simulink model "Citation_Sim"  (R2019b)
settings: Solver=VariableStepAuto  StartTime=0.0  StopTime=10.0  RelTol=1e-3
values from neighbouring files (symbols this model uses):
  A = [-0.0151 -60.5651 0 -32.174 ... (first row only)    [UnstableAircraft.m]    (also in VincentMPCCode.m = [0 0 1 0; 0 0 0 1; -(Ks+Kus)/Mus Ks/Mus -Bs/Mus Bs/Mus; Ks/M; qpsoft.m = [           A,             minusones; scmpc4.m = [A;Su(iymax,:)]; scmpcnl2.m = [A;Su(iymax,:)])
  B = [-2.516 -13.136 ... (first row only)    [UnstableAircraft.m]    (also in VincentMPCCode.m = [0 0; 0 0; -1/Mus Kus/Mus; 1/Ms 0]; qpsoft.m = [         B; scmpc4.m = SuTQ*Su+diag(R); scmpcnl2.m = SuTQ*Su+diag(R))
  C = [0 1 0 0 ... (first row only)    [UnstableAircraft.m]    (also in VincentMPCCode.m = [1 0 0 0; -1 1 0 0; 0 0 1 0; 0 0 0 1])
  D = [0 0 ... (first row only)    [UnstableAircraft.m]    (also in VincentMPCCode.m = [0 -1; 0 0; 0 0; 0 0])
libraries: mpclib x1
settings Model: Creator=kieran  LastModifiedBy=kieran

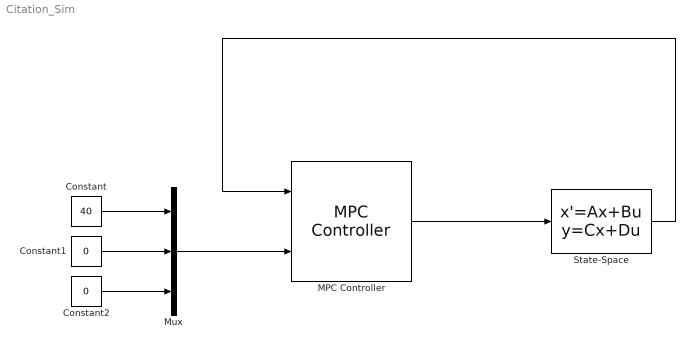
== system Citation_Sim ==
  Constant : Constant  Value=40
  Constant1 : Constant  Value=0
  Constant2 : Constant  Value=0
  MPC Controller : mpclib/MPC Controller  SCDEnableBlockLinearizationSpecification=on  is_multiple=0  enable_value=0  return_u0=off  updateMPCinCallerWorkspace=on  md_inport=off  mv_inport=off  uref_inport=off  return_cost=off  return_mvseq=off  return_qpstatus=off  return_xseq=off  return_state=off  return_ovseq=off  state_inport=off  umin_inport=off  umax_inport=off  ymin_inport=off  ymax_inport=off  cc_inport=off  ywt_inport=off  uwt_inport=off  duwt_inport=off  rhoeps_inport=off  pm_inport=off  MaximumP=10  HorizonChoice=FixedHorizon  n_ts=1  n_p=10  n_mv=1  n_md=1  n_ud=0  n_mo=1  n_uo=0  BlockDataType=double  SampleTimeInherited=off  switch_inport=off
  Mux : Mux  Inputs=3
  State-Space : StateSpace  A=A  B=B  C=C  D=D  InitialCondition=0
  wires:
  MPC Controller/1 -> State-Space/1
  State-Space/1 -> MPC Controller/1
  Constant/1 -> Mux/1
  Constant1/1 -> Mux/2
  Constant2/1 -> Mux/3
  Mux/1 -> MPC Controller/2
